simulink model "RollReducedModel_New_R2019a"  (R2019a)
settings: Solver=VariableStepAuto  StartTime=0.0  StopTime=10.0  RelTol=1e-3
PreLoadFcn:
  | JointParameters
values from neighbouring files (symbols this model uses):
  b = 0.1    [JointParameters.m]
  B_l = 0.5    [JointParameters.m]
  B_u = 0.5    [JointParameters.m]
  CurrThrust = 60    [JointParameters.m]
  g = 9.81    [JointParameters.m]
  J_l = 0.071440709    [JointParameters.m]
  J_u = 0.049103    [JointParameters.m]
  k = 0.13    [JointParameters.m]
  L_cg_l = 0.102366    [JointParameters.m]
  L_cg_u = 0.066301    [JointParameters.m]
  L_l = 0.223793    [JointParameters.m]
  L_u = 0.227293    [JointParameters.m]
  mass_l = 2.495    [JointParameters.m]
  mass_u = 2.024    [JointParameters.m]
  MotorSaturation = 40    [JointParameters.m]
undefined symbols (not defined in the file or in its folder): Jroll, Lr, mr, rr
libraries: simulink x6
settings Model: Creator=user  LastModifiedBy=user
settings DebuggingCC: UnconnectedInputMsg=none  UnconnectedOutputMsg=none  UnconnectedLineMsg=none
settings ModelReferenceCC: EnableRefExpFcnMdlSchedulingChecks=off
settings RTWCC: Description=Generic Real-Time Target

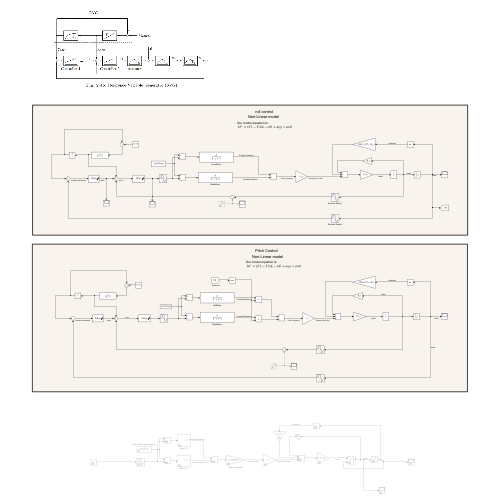
[thumbnail: Simulink's stored preview of the top-level diagram]
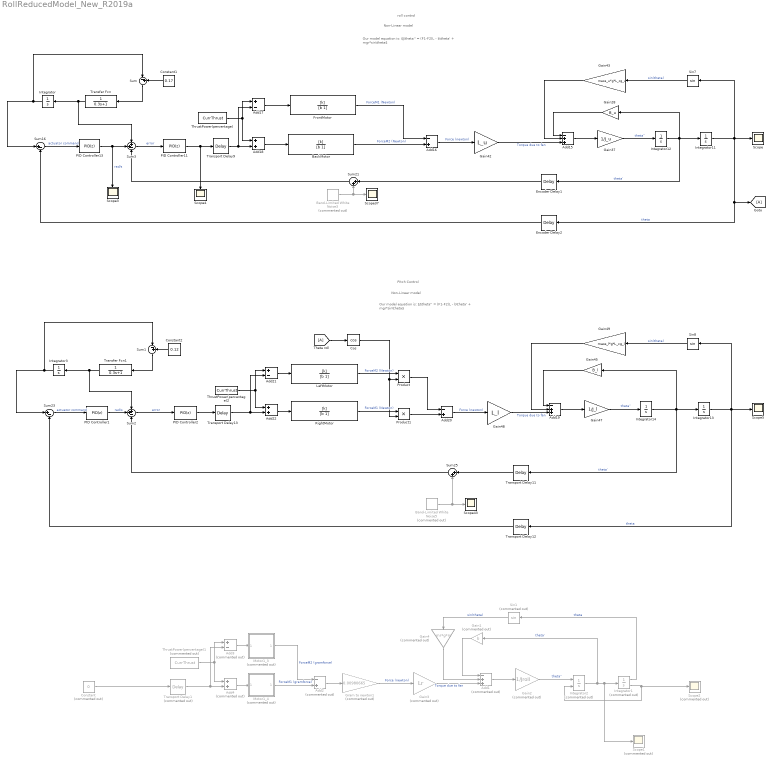
== system RollReducedModel_New_R2019a ==
  note: Our model equation is:
      | $J\theta'' = (F1-F2)L - b\theta' + mgr*sin\theta$
  note: Our model equation is:
      | $J\theta'' = (F1-F2)L - b\theta' + mgr*sin\theta$
  note: Non-Linear model
  note: Pitch Control
  note: Non-Linear model
  note: roll control
  Add1 : Sum  Commented=on  Inputs=-++
  Add15 : Sum  Inputs=-++
  Add16 : Sum  Inputs=-+
  Add17 : Sum  Inputs=+-
  Add18 : Sum
  Add19 : Sum  Inputs=-++
  Add2 : Sum  Commented=on  Inputs=-+
  Add20 : Sum  Inputs=-+
  Add21 : Sum  Inputs=+-
  Add22 : Sum
  Add3 : Sum  Commented=on  Inputs=+-
  Add4 : Sum  Commented=on
  BackMotor : TransferFcn  Numerator=[k]  Denominator=[b 1]
  Band-Limited White Noise3 : simulink/Sources/Band-Limited White Noise  Commented=on  Cov=0.000005  Ts=0.0225  seed=[23341]
  Band-Limited White Noise5 : simulink/Sources/Band-Limited White Noise  Commented=on  Cov=0.000005  Ts=0.0225  seed=[23341]
  Constant : Constant  Commented=on  Value=0
  Constant1 : Constant  Value=0.17
  Constant2 : Constant  Value=0.12
  Cos : Trigonometry  Operator=cos
  Encoder Delay1 : TransportDelay  DelayTime=0.0225
  Encoder Delay2 : TransportDelay  DelayTime=0.0225
  FrontMotor : TransferFcn  Numerator=[k]  Denominator=[b 1]
  Gain1 : Gain  Commented=on  Gain=b
  Gain2 : Gain  Commented=on  Gain=1/Jroll
  Gain28 : Gain  Gain=B_u
  Gain3 : Gain  Commented=on  Gain=Lr
  Gain37 : Gain  Gain=1/J_u
  Gain4 : Gain  Commented=on  Gain=mr*g*rr
  Gain42 : Gain  Gain=L_u
  Gain43 : Gain  Gain=mass_u*g*L_cg_u
  Gain45 : Gain  Gain=B_l
  Gain47 : Gain  Gain=1/J_l
  Gain48 : Gain  Gain=L_l
  Gain49 : Gain  Gain=mass_l*g*L_cg_l
  Gram to newton1 : Gain  Commented=on  Gain=0.00980665
  Integrator{,3,12,14} (4 alike) : Integrator
  Integrator1 : Integrator  Commented=on  LimitOutput=on  UpperSaturationLimit=0.7  LowerSaturationLimit=-0.7  ShowSaturationPort=on
  Integrator11 : Integrator  LimitOutput=on  UpperSaturationLimit=0.4  LowerSaturationLimit=-0.33
  Integrator13 : Integrator  LimitOutput=on  UpperSaturationLimit=0.27  LowerSaturationLimit=-0.37
  Integrator2 : Integrator  Commented=on  ExternalReset=level hold
  LeftMotor : TransferFcn  Numerator=[k]  Denominator=[b 1]
  Motor1_3 : Subsystem  Commented=on
      mask Display: image('2200kv.jpg');
  Motor1_4 : Subsystem  Commented=on
      mask Display: image('2200kv.jpg');
  PID Controller1 : simulink/Continuous/PID Controller  Controller=PID  Form=Parallel  TimeDomain=Discrete-time  SampleTime=0.005  IntegratorMethod=Forward Euler  ControllerParametersSource=internal  P=2  I=2  D=0  N=10  UseFilter=on  TunerSelectOption=Transfer Function Based (PID Tuner App)  InitialConditionSource=internal  InitialConditionForIntegrator=0  InitialConditionForFilter=0  DifferentiatorICPrevScaledInput=0  ExternalReset=none  TrackingMode=off  Kt=1  LimitOutput=on  UpperSaturationLimit=0.17  LowerSaturationLimit=-0.17  LinearizeAsGain=on  AntiWindupMode=clamping  Kb=1  POutMin=[]  POutMax=[]  IOutMin=[]  IOutMax=[]  DOutMin=[]  DOutMax=[]  NOutMin=[]  NOutMax=[]  SumOutMin=[]  SumOutMax=[]  SaturationOutMin=[]  SaturationOutMax=[]  PParamMin=[]  PParamMax=[]  IParamMin=[]  IParamMax=[]  DParamMin=[]  DParamMax=[]  NParamMin=[]  NParamMax=[]  KbParamMin=[]  KbParamMax=[]  KtParamMin=[]  KtParamMax=[]  KbOutMin=[]  KbOutMax=[]  KtOutMin=[]  KtOutMax=[]  IntegratorOutMin=[]  IntegratorOutMax=[]  FilterOutMin=[]  FilterOutMax=[]  SumI1OutMin=[]  SumI1OutMax=[]  SumI2OutMin=[]  SumI2OutMax=[]  SumI3OutMin=[]  SumI3OutMax=[]  SumI4OutMin=[]  SumI4OutMax=[]  SumDOutMin=[]  SumDOutMax=[]  DifferentiatorOutMin=[]  DifferentiatorOutMax=[]  FilterDiffOutCoefMin=[]  FilterDiffOutCoefMax=[]  ReciprocalOutMin=[]  ReciprocalOutMax=[]  SumDenOutMin=[]  SumDenOutMax=[]  SumNumOutMin=[]  SumNumOutMax=[]  DivideOutMin=[]  DivideOutMax=[]  IntegratorContinuousStateAttributes=''  IntegratorStateMustResolveToSignalObject=off  IntegratorRTWStateStorageClass=Auto  FilterContinuousStateAttributes=''  FilterStateMustResolveToSignalObject=off  FilterRTWStateStorageClass=Auto  ParallelPVariant=InternalParameters  IdealPVariant=Disabled  IVariant=InternalParameters  DVariant=InternalParameters  IntegratorVariant=Discrete  SatVariant=Enabled  AWVariant=DiscClampingParallel  PCopyVariant=Disabled  TRVariant=Disabled  FdbkBlocksVariant=Forward  IdealPFdbkVariant=Disabled  SatFdbkVariant=Disabled  DerivativeFilterVariant=ForwardEulerFilter  NVariant=InternalParameters  NCopyVariant=Disabled  FilterICVariant=InternalICsFilter  IntegratorICVariant=InternalICs  ExternalResetVariant=Disabled  TRSumVariant=Passthrough  SumFdbkVariant=Disabled  SumVariant=Sum_PID
  PID Controller11 : simulink/Continuous/PID Controller  Controller=PID  Form=Parallel  TimeDomain=Discrete-time  SampleTime=0.005  IntegratorMethod=Forward Euler  ControllerParametersSource=internal  P=500  I=100  D=0  N=10  UseFilter=on  TunerSelectOption=Transfer Function Based (PID Tuner App)  InitialConditionSource=internal  InitialConditionForIntegrator=0  InitialConditionForFilter=0  DifferentiatorICPrevScaledInput=0  ExternalReset=none  TrackingMode=off  Kt=1  LimitOutput=on  UpperSaturationLimit=MotorSaturation  LowerSaturationLimit=-MotorSaturation  LinearizeAsGain=on  AntiWindupMode=clamping  Kb=1  POutMin=[]  POutMax=[]  IOutMin=[]  IOutMax=[]  DOutMin=[]  DOutMax=[]  NOutMin=[]  NOutMax=[]  SumOutMin=[]  SumOutMax=[]  SaturationOutMin=[]  SaturationOutMax=[]  PParamMin=[]  PParamMax=[]  IParamMin=[]  IParamMax=[]  DParamMin=[]  DParamMax=[]  NParamMin=[]  NParamMax=[]  KbParamMin=[]  KbParamMax=[]  KtParamMin=[]  KtParamMax=[]  KbOutMin=[]  KbOutMax=[]  KtOutMin=[]  KtOutMax=[]  IntegratorOutMin=[]  IntegratorOutMax=[]  FilterOutMin=[]  FilterOutMax=[]  SumI1OutMin=[]  SumI1OutMax=[]  SumI2OutMin=[]  SumI2OutMax=[]  SumI3OutMin=[]  SumI3OutMax=[]  SumI4OutMin=[]  SumI4OutMax=[]  SumDOutMin=[]  SumDOutMax=[]  DifferentiatorOutMin=[]  DifferentiatorOutMax=[]  FilterDiffOutCoefMin=[]  FilterDiffOutCoefMax=[]  ReciprocalOutMin=[]  ReciprocalOutMax=[]  SumDenOutMin=[]  SumDenOutMax=[]  SumNumOutMin=[]  SumNumOutMax=[]  DivideOutMin=[]  DivideOutMax=[]  IntegratorContinuousStateAttributes=''  IntegratorStateMustResolveToSignalObject=off  IntegratorRTWStateStorageClass=Auto  FilterContinuousStateAttributes=''  FilterStateMustResolveToSignalObject=off  FilterRTWStateStorageClass=Auto  ParallelPVariant=InternalParameters  IdealPVariant=Disabled  IVariant=InternalParameters  DVariant=InternalParameters  IntegratorVariant=Discrete  SatVariant=Enabled  AWVariant=DiscClampingParallel  PCopyVariant=Disabled  TRVariant=Disabled  FdbkBlocksVariant=Forward  IdealPFdbkVariant=Disabled  SatFdbkVariant=Disabled  DerivativeFilterVariant=ForwardEulerFilter  NVariant=InternalParameters  NCopyVariant=Disabled  FilterICVariant=InternalICsFilter  IntegratorICVariant=InternalICs  ExternalResetVariant=Disabled  TRSumVariant=Passthrough  SumFdbkVariant=Disabled  SumVariant=Sum_PID
  PID Controller13 : simulink/Continuous/PID Controller  Controller=PID  Form=Parallel  TimeDomain=Discrete-time  SampleTime=0.005  IntegratorMethod=Forward Euler  ControllerParametersSource=internal  P=2  I=2  D=0  N=10  UseFilter=on  TunerSelectOption=Transfer Function Based (PID Tuner App)  InitialConditionSource=internal  InitialConditionForIntegrator=0  InitialConditionForFilter=0  DifferentiatorICPrevScaledInput=0  ExternalReset=none  TrackingMode=off  Kt=1  LimitOutput=on  UpperSaturationLimit=0.17  LowerSaturationLimit=-0.17  LinearizeAsGain=on  AntiWindupMode=clamping  Kb=1  POutMin=[]  POutMax=[]  IOutMin=[]  IOutMax=[]  DOutMin=[]  DOutMax=[]  NOutMin=[]  NOutMax=[]  SumOutMin=[]  SumOutMax=[]  SaturationOutMin=[]  SaturationOutMax=[]  PParamMin=[]  PParamMax=[]  IParamMin=[]  IParamMax=[]  DParamMin=[]  DParamMax=[]  NParamMin=[]  NParamMax=[]  KbParamMin=[]  KbParamMax=[]  KtParamMin=[]  KtParamMax=[]  KbOutMin=[]  KbOutMax=[]  KtOutMin=[]  KtOutMax=[]  IntegratorOutMin=[]  IntegratorOutMax=[]  FilterOutMin=[]  FilterOutMax=[]  SumI1OutMin=[]  SumI1OutMax=[]  SumI2OutMin=[]  SumI2OutMax=[]  SumI3OutMin=[]  SumI3OutMax=[]  SumI4OutMin=[]  SumI4OutMax=[]  SumDOutMin=[]  SumDOutMax=[]  DifferentiatorOutMin=[]  DifferentiatorOutMax=[]  FilterDiffOutCoefMin=[]  FilterDiffOutCoefMax=[]  ReciprocalOutMin=[]  ReciprocalOutMax=[]  SumDenOutMin=[]  SumDenOutMax=[]  SumNumOutMin=[]  SumNumOutMax=[]  DivideOutMin=[]  DivideOutMax=[]  IntegratorContinuousStateAttributes=''  IntegratorStateMustResolveToSignalObject=off  IntegratorRTWStateStorageClass=Auto  FilterContinuousStateAttributes=''  FilterStateMustResolveToSignalObject=off  FilterRTWStateStorageClass=Auto  ParallelPVariant=InternalParameters  IdealPVariant=Disabled  IVariant=InternalParameters  DVariant=InternalParameters  IntegratorVariant=Discrete  SatVariant=Enabled  AWVariant=DiscClampingParallel  PCopyVariant=Disabled  TRVariant=Disabled  FdbkBlocksVariant=Forward  IdealPFdbkVariant=Disabled  SatFdbkVariant=Disabled  DerivativeFilterVariant=ForwardEulerFilter  NVariant=InternalParameters  NCopyVariant=Disabled  FilterICVariant=InternalICsFilter  IntegratorICVariant=InternalICs  ExternalResetVariant=Disabled  TRSumVariant=Passthrough  SumFdbkVariant=Disabled  SumVariant=Sum_PID
  PID Controller2 : simulink/Continuous/PID Controller  Controller=PID  Form=Parallel  TimeDomain=Discrete-time  SampleTime=0.005  IntegratorMethod=Forward Euler  ControllerParametersSource=internal  P=500  I=100  D=0  N=10  UseFilter=on  TunerSelectOption=Transfer Function Based (PID Tuner App)  InitialConditionSource=internal  InitialConditionForIntegrator=0  InitialConditionForFilter=0  DifferentiatorICPrevScaledInput=0  ExternalReset=none  TrackingMode=off  Kt=1  LimitOutput=on  UpperSaturationLimit=MotorSaturation  LowerSaturationLimit=-MotorSaturation  LinearizeAsGain=on  AntiWindupMode=clamping  Kb=1  POutMin=[]  POutMax=[]  IOutMin=[]  IOutMax=[]  DOutMin=[]  DOutMax=[]  NOutMin=[]  NOutMax=[]  SumOutMin=[]  SumOutMax=[]  SaturationOutMin=[]  SaturationOutMax=[]  PParamMin=[]  PParamMax=[]  IParamMin=[]  IParamMax=[]  DParamMin=[]  DParamMax=[]  NParamMin=[]  NParamMax=[]  KbParamMin=[]  KbParamMax=[]  KtParamMin=[]  KtParamMax=[]  KbOutMin=[]  KbOutMax=[]  KtOutMin=[]  KtOutMax=[]  IntegratorOutMin=[]  IntegratorOutMax=[]  FilterOutMin=[]  FilterOutMax=[]  SumI1OutMin=[]  SumI1OutMax=[]  SumI2OutMin=[]  SumI2OutMax=[]  SumI3OutMin=[]  SumI3OutMax=[]  SumI4OutMin=[]  SumI4OutMax=[]  SumDOutMin=[]  SumDOutMax=[]  DifferentiatorOutMin=[]  DifferentiatorOutMax=[]  FilterDiffOutCoefMin=[]  FilterDiffOutCoefMax=[]  ReciprocalOutMin=[]  ReciprocalOutMax=[]  SumDenOutMin=[]  SumDenOutMax=[]  SumNumOutMin=[]  SumNumOutMax=[]  DivideOutMin=[]  DivideOutMax=[]  IntegratorContinuousStateAttributes=''  IntegratorStateMustResolveToSignalObject=off  IntegratorRTWStateStorageClass=Auto  FilterContinuousStateAttributes=''  FilterStateMustResolveToSignalObject=off  FilterRTWStateStorageClass=Auto  ParallelPVariant=InternalParameters  IdealPVariant=Disabled  IVariant=InternalParameters  DVariant=InternalParameters  IntegratorVariant=Discrete  SatVariant=Enabled  AWVariant=DiscClampingParallel  PCopyVariant=Disabled  TRVariant=Disabled  FdbkBlocksVariant=Forward  IdealPFdbkVariant=Disabled  SatFdbkVariant=Disabled  DerivativeFilterVariant=ForwardEulerFilter  NVariant=InternalParameters  NCopyVariant=Disabled  FilterICVariant=InternalICsFilter  IntegratorICVariant=InternalICs  ExternalResetVariant=Disabled  TRSumVariant=Passthrough  SumFdbkVariant=Disabled  SumVariant=Sum_PID
  Product : Product
  Product1 : Product
  RightMotor : TransferFcn  Numerator=[k]  Denominator=[b 1]
  Scope{,3..5,37,43} (6 alike) : Scope
  Scope1 : Scope  Commented=on
  Scope2 : Scope  Commented=on
  Sin1 : Trigonometry  Commented=on
  Sin7 : Trigonometry
  Sin8 : Trigonometry
  Sum : Sum  Inputs=|-+
  Sum1 : Sum  Inputs=|-+
  Sum16 : Sum  Inputs=|+-
  Sum2 : Sum  Inputs=++-
  Sum21 : Sum  Inputs=|++
  Sum23 : Sum  Inputs=|+-
  Sum25 : Sum  Inputs=|++
  Sum3 : Sum  Inputs=++-
  ThrustPower(percentage) : Constant  Value=CurrThrust
  ThrustPower(percentage)1 : Constant  Commented=on  Value=CurrThrust
  ThrustPower(percentage)2 : Constant  Value=CurrThrust
  Transfer Fcn : TransferFcn  Denominator=[0.3 1]
  Transfer Fcn1 : TransferFcn  Denominator=[0.3 1]
  Transport Delay1 : TransportDelay  Commented=on  DelayTime=0.05
  Transport Delay11 : TransportDelay  DelayTime=0.0225
  Transport Delay12 : TransportDelay  DelayTime=0.0225
  Transport Delay13 : TransportDelay  DelayTime=0.05
  Transport Delay9 : TransportDelay  DelayTime=0.005
  wires:
  Cos/1 -> Product1/2, Product/2
  Add19/1 -> Gain47/1
  ThrustPower(percentage)2/1 -> Add22/1, Add21/1
  Product1/1 -> Add20/2
  Gain49/1 -> Add19/2
  Gain45/1 -> Add19/1
  Gain37/1 -> Integrator12/1  "theta''"
  Integrator11/1 -> Encoder Delay2/1, [A], Scope/1, Sin7/1  "theta"
  Sum25/1 -> Sum2/3
  Sum2/1 -> PID Controller2/1  "error"
  Integrator14/1 -> Transport Delay11/1, Integrator13/1, Gain45/1  "theta'"
  Band-Limited White Noise5/1 -> Scope43/1, Sum25/2
  Add20/1 -> Gain48/1  "Force (newton)"
  Gain48/1 -> Add19/3  "Torque due to fan"
  PID Controller1/1 -> Sum2/2  "rad/s"
  FrontMotor/1 -> Add16/1  "ForceM1 (Newton)"
  Integrator13/1 -> Transport Delay12/1, Scope5/1, Sin8/1  "theta"
  LeftMotor/1 -> Product/1  "ForceM2 (Newton)"
  Gain47/1 -> Integrator14/1  "theta''"
  Add21/1 -> LeftMotor/1
  Product/1 -> Add20/1
  ThrustPower(percentage)/1 -> Add18/1, Add17/1
  BackMotor/1 -> Add16/2  "ForceM2 (Newton)"
  RightMotor/1 -> Product1/1  "ForceM1 (Newton)"
  Sum21/1 -> Sum3/3
  Add18/1 -> BackMotor/1
  PID Controller2/1 -> Transport Delay13/1
  Sum23/1 -> PID Controller1/1  "actuator command"
  Add22/1 -> RightMotor/1
  Integrator3/1 -> Sum23/1, Sum1/1
  PID Controller13/1 -> Scope3/1, Sum3/2  "rad/s"
  Sin7/1 -> Gain43/1  "sin(theta)"
  Add16/1 -> Gain42/1  "Force (newton)"
  Gain42/1 -> Add15/3  "Torque due to fan"
  Add17/1 -> FrontMotor/1
  Gain28/1 -> Add15/1
  Gain43/1 -> Add15/2
  Add15/1 -> Gain37/1
  Sum3/1 -> PID Controller11/1  "error"
  Band-Limited White Noise3/1 -> Sum21/2, Scope37/1
  Integrator12/1 -> Encoder Delay1/1, Integrator11/1, Gain28/1  "theta'"
  Sum16/1 -> PID Controller13/1  "actuator command"
  Sin8/1 -> Gain49/1  "sin(theta)"
  [A] -> Cos/1
  Integrator1/2 -> Integrator2/2, Scope2/1
  Integrator2/1 -> Gain1/1, Scope1/1, Integrator1/1  "theta'"
  Transport Delay1/1 -> Add4/2, Add3/2
  Add1/1 -> Gain2/1
  Gain4/1 -> Add1/2
  Gain1/1 -> Add1/1
  Add3/1 -> Motor1_3/1(MotorPercentage)
  Gain3/1 -> Add1/3  "Torque due to fan"
  Gram to newton1/1 -> Gain3/1  "Force (newton)"
  Sin1/1 -> Gain4/1  "sin(theta)"
  Add4/1 -> Motor1_4/1(MotorPercentage)
  Motor1_4/1(MotorForce) -> Add2/2  "ForceM1 (gramforce)"
  ThrustPower(percentage)1/1 -> Add3/1, Add4/1
  Motor1_3/1(MotorForce) -> Add2/1  "ForceM2 (gramforce)"
  Add2/1 -> Gram to newton1/1
  Integrator1/1 -> Sin1/1  "theta"
  Gain2/1 -> Integrator2/1  "theta''"
  Constant/1 -> Transport Delay1/1
  Integrator/1 -> Sum16/1, Sum/1
  Transfer Fcn/1 -> Sum3/1, Integrator/1
  Constant1/1 -> Sum/2
  Sum/1 -> Transfer Fcn/1
  Sum1/1 -> Transfer Fcn1/1
  Constant2/1 -> Sum1/2
  Transfer Fcn1/1 -> Sum2/1, Integrator3/1
  PID Controller11/1 -> Scope4/1, Transport Delay9/1
  Transport Delay9/1 -> Add17/2, Add18/2
  Encoder Delay1/1 -> Sum21/1
  Encoder Delay2/1 -> Sum16/2
  Transport Delay13/1 -> Add22/2, Add21/2
  Transport Delay11/1 -> Sum25/1
  Transport Delay12/1 -> Sum23/2

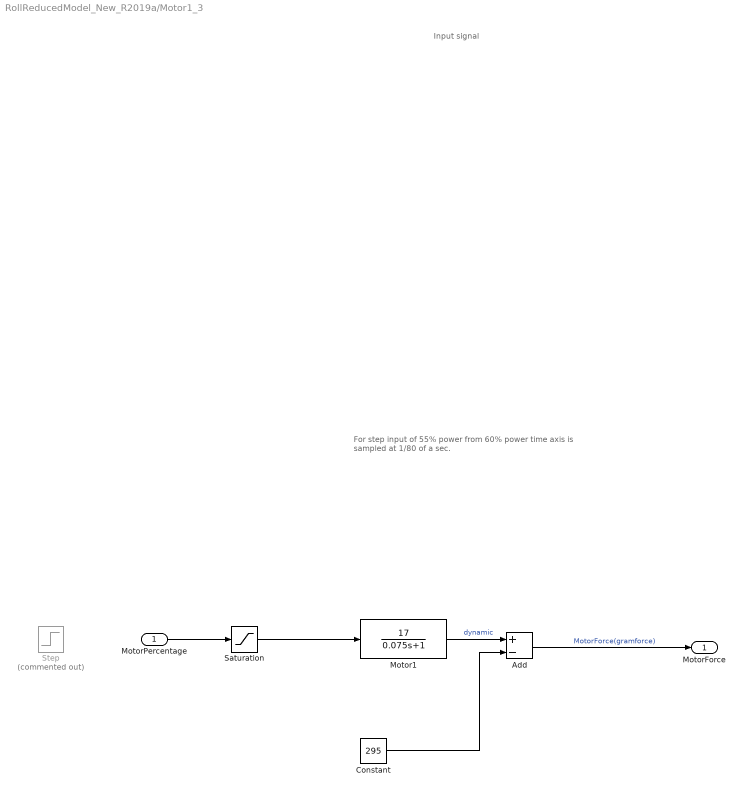
== system RollReducedModel_New_R2019a/Motor1_3 ==
  note: For step input of 55% power from 60% power
      | time axis is sampled at 1/80 of a sec.
  note: Input signal
  MotorPercentage : Inport
  Add : Sum  Inputs=+-
  Constant : Constant  Value=295
  Motor1 : TransferFcn  Numerator=[17]  Denominator=[0.075 1]
  Saturation : Saturate  UpperLimit=100  LowerLimit=0
  Step : Step  Commented=on  Time=2  Before=60  After=55  SampleTime=0
  MotorForce : Outport
  wires:
  Constant/1 -> Add/2
  Motor1/1 -> Add/1  "dynamic"
  Add/1 -> MotorForce/1  "MotorForce(gramforce)"
  MotorPercentage/1 -> Saturation/1
  Saturation/1 -> Motor1/1

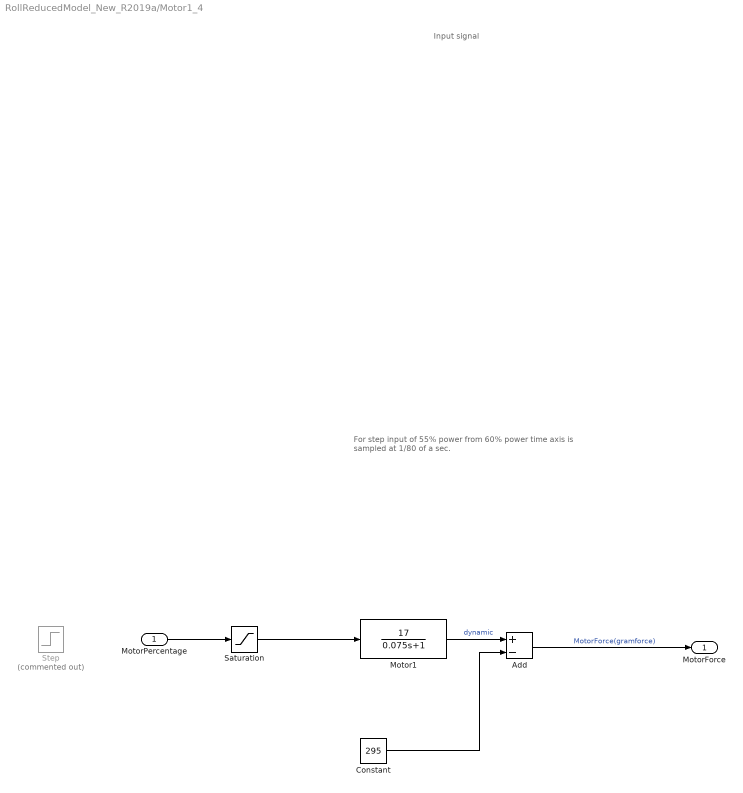
== system RollReducedModel_New_R2019a/Motor1_4 ==
  note: Input signal
  note: For step input of 55% power from 60% power
      | time axis is sampled at 1/80 of a sec.
  MotorPercentage : Inport
  Add : Sum  Inputs=+-
  Constant : Constant  Value=295
  Motor1 : TransferFcn  Numerator=[17]  Denominator=[0.075 1]
  Saturation : Saturate  UpperLimit=100  LowerLimit=0
  Step : Step  Commented=on  Time=2  Before=60  After=55  SampleTime=0
  MotorForce : Outport
  wires:
  Saturation/1 -> Motor1/1
  MotorPercentage/1 -> Saturation/1
  Add/1 -> MotorForce/1  "MotorForce(gramforce)"
  Motor1/1 -> Add/1  "dynamic"
  Constant/1 -> Add/2
